simulink model "testmodel2017b"  (R2017b)
settings: Solver=FixedStepDiscrete  StartTime=0.0  StopTime=10000  FixedStep=srate  RelTol=1e-3
PreLoadFcn:
  | model_startup;
model workspace (MAT data in the model file):
  CD_IFBK_GAIN = Simulink.Parameter
  CD_IFBK_GAIN.Value = 0.00279947916667
  CD_IFBK_GAIN.DataType = 'single'
  CD_IFBK_GAIN.Dimensions = [1 1]
  CD_INTEGRATOR_RESET_I = Simulink.Parameter
  CD_INTEGRATOR_RESET_I.Value = 0.01
  CD_INTEGRATOR_RESET_I.DataType = 'single'
  CD_INTEGRATOR_RESET_I.Dimensions = [1 1]
  CD_PRECISION_REF_NOM = Simulink.Parameter
  CD_PRECISION_REF_NOM.Value = 511
  CD_PRECISION_REF_NOM.DataType = 'single'
  CD_PRECISION_REF_NOM.Dimensions = [1 1]
  CD_SOLENOID_RES = Simulink.Parameter
  CD_SOLENOID_RES.Value = 6.1803
  CD_SOLENOID_RES.DataType = 'single'
  CD_SOLENOID_RES.Dimensions = [1 1]
  CD_VBATTERY_GAIN = Simulink.Parameter
  CD_VBATTERY_GAIN.Value = 0.0293360157816
  CD_VBATTERY_GAIN.DataType = 'single'
  CD_VBATTERY_GAIN.Dimensions = [1 1]
  CD_VBATTERY_NOM = Simulink.Parameter
  CD_VBATTERY_NOM.Value = 13.5
  CD_VBATTERY_NOM.DataType = 'single'
  CD_VBATTERY_NOM.Dimensions = [1 1]
  OnPower = Simulink.Signal
  OnPower.DataType = 'boolean'
  OnPower.Dimensions = -1
  OnPower.DimensionsMode = 'auto'
  OnPower.Complexity = 'auto'
  OnPower.SampleTime = -1
  OnPower.SamplingMode = 'auto'
  numOutputs = 6
  srate = 0.01
undefined symbols (not defined in the file): CMD_INVERTER_GOTO_OPERATIONAL, CMD_INVERTER_GOTO_READY, CMD_INVERTER_GOTO_STOP, CMD_INVERTER_RUN_FWD, INVERTER_CONNECTED, INVERTER_OPERATIONAL, INVERTER_READY, INVERTER_RUN_FWD, INVERTER_STOP
libraries: simulink x8
CloseFcn:
  | model_end;
settings Model: Creator=cswenson  LastModifiedBy=mmaffeo
settings DataIOCC: SaveOutput=off  SaveTime=off
settings OptimizationCC: DefaultParameterBehavior=Inlined  InlineInvariantSignals=on  EnhancedBackFolding=on  PassReuseOutputArgsAs=Individual arguments  LifeSpan=inf  OptimizeBlockOrder=speed  DifferentSizesBufferReuse=on
settings DebuggingCC: SignalInfNanChecking=error  SignalRangeChecking=error  ReadBeforeWriteMsg=EnableAllAsError  WriteAfterWriteMsg=EnableAllAsError  WriteAfterReadMsg=EnableAllAsError  AlgebraicLoopMsg=error  ArtificialAlgebraicLoopMsg=error  SaveWithParameterizedLinksMsg=error  BlockPriorityViolationMsg=error  SolverPrmCheckMsg=error  InheritedTsInSrcMsg=error  SigSpecEnsureSampleTimeMsg=error  CheckMatrixSingularityMsg=error  IntegerOverflowMsg=error  ParameterUnderflowMsg=warning  ParameterTunabilityLossMsg=error  UnderSpecifiedDataTypeMsg=error  UnnecessaryDatatypeConvMsg=warning  VectorMatrixConversionMsg=error  FcnCallInpInsideContextMsg=warning  UnconnectedInputMsg=error  UnconnectedOutputMsg=error  UnconnectedLineMsg=error  SFcnCompatibilityMsg=error  UniqueDataStoreMsg=error  BusObjectLabelMismatch=error  RootOutportRequireBusObject=error  AssertControl=DisableAll  ModelReferenceIOMsg=error  ModelReferenceIOMismatchMessage=error  UnknownTsInhSupMsg=error  ModelReferenceDataLoggingMessage=error  StateNameClashWarn=warning  SFUnexpectedBacktrackingDiag=warning  SFNoUnconditionalDefaultTransitionDiag=warning  SFExecutionAtInitializationDiag=none
settings HardwareCC: ProdBitPerPointer=32  ProdBitPerSizeT=32  ProdBitPerPtrDiffT=32  ProdLargestAtomicInteger=Long  ProdLargestAtomicFloat=Double  ProdWordSize=32  ProdHWDeviceType=ARM Compatible->ARM Cortex  TargetBitPerPointer=64  TargetBitPerSizeT=64  TargetBitPerPtrDiffT=64  TargetLongLongMode=on  TargetIntDivRoundTo=Zero  TargetEndianess=LittleEndian  TargetWordSize=64  TargetHWDeviceType=MATLAB Host
settings ModelReferenceCC: PropagateSignalLabelsOutOfModel=off
settings SFSimCC: SimUserSources=SendMsgNow_Blank.cpp  SimUserIncludeDirs=functions  MATLABDynamicMemAlloc=off
settings SFSimCC: SimCustomHeaderCode=|
  | #include "SendMsgNow.h"
  | #define uint8_t unsigned char
settings RTWCC: SystemTargetFile=bobcat_ert.tlc  GenCodeOnly=on  GenerateMakefile=off  TemplateMakefile=ert_default_tmf  Description=Bobcat Embedded Target derived from RTW-EC  GenerateReport=on  RTWVerbose=off  IncludeHyperlinkInReport=on  LaunchReport=on  PortableWordSizes=on  TargetLang=C++  GenerateTraceInfo=on  GenerateTraceReport=on  GenerateTraceReportSl=on  GenerateTraceReportSf=on  GenerateTraceReportEml=on  GenerateCodeMetricsReport=on  GenerateCodeReplacementReport=on
settings RTWCC: CustomHeaderCode=|
  | #include "cdata.h"
  | #include "ap_can.h"
  | #include "SendMsgNow.h"
  | #include "ap_eeprom.h"
  | #include "ap_bservice_CAN04.h"
settings CodeAppCC: ForceParamTrailComments=on  IgnoreCustomStorageClasses=off  IgnoreTestpoints=on  MangleLength=4  StateflowObjectComments=on  InternalIdentifier=Classic  ReqsInCode=on
settings STFCustomTargetCC: MultiwordLength=256  IncludeMdlTerminateFcn=off  CombineOutputUpdateFcns=on  ERTCustomFileBanners=on  SupportNonFinite=off  SupportComplex=off  SupportNonInlinedSFcns=off  MATLABClassNameForMDSCustomization=Simulink.SoftwareTarget.ERTCustomization  GRTInterface=off  SystemTargetFile=bobcat_ert.tlc
settings ERTTargetCC: ParMdlRefBuildCompliant=off  CompOptLevelCompliant=off  ConcurrentExecutionCompliant=off  IncludeMdlTerminateFcn=off  SupportNonFinite=off  SupportComplex=off  SupportContinuousTime=on  RemoveResetFunc=off  ModelStepFunctionPrototypeControlCompliant=off  CPPClassGenCompliant=off  UseToolchainInfoCompliant=off  InlinedParameterPlacement=NonHierarchical  ERTSrcFileBannerTemplate=bobcat_ert_template.cgt  ERTHdrFileBannerTemplate=bobcat_ert_template.cgt  ERTDataSrcFileTemplate=bobcat_ert_template.cgt  ERTDataHdrFileTemplate=bobcat_ert_template.cgt  ERTCustomFileTemplate=bobcat_file_process.tlc  PreserveExpressionOrder=on  PreserveIfCondition=on  ConvertIfToSwitch=off  SuppressUnreachableDefaultCases=off
settings ConfigComp: CovScope=ReferencedModels  CovIncludeTopModel=off  CovMetricSettings=dw  CovHtmlReporting=on  CovSaveCumulativeToWorkspaceVar=on  CovSaveSingleToWorkspaceVar=on  CovExternalEMLEnable=off  CovSFcnEnable=off

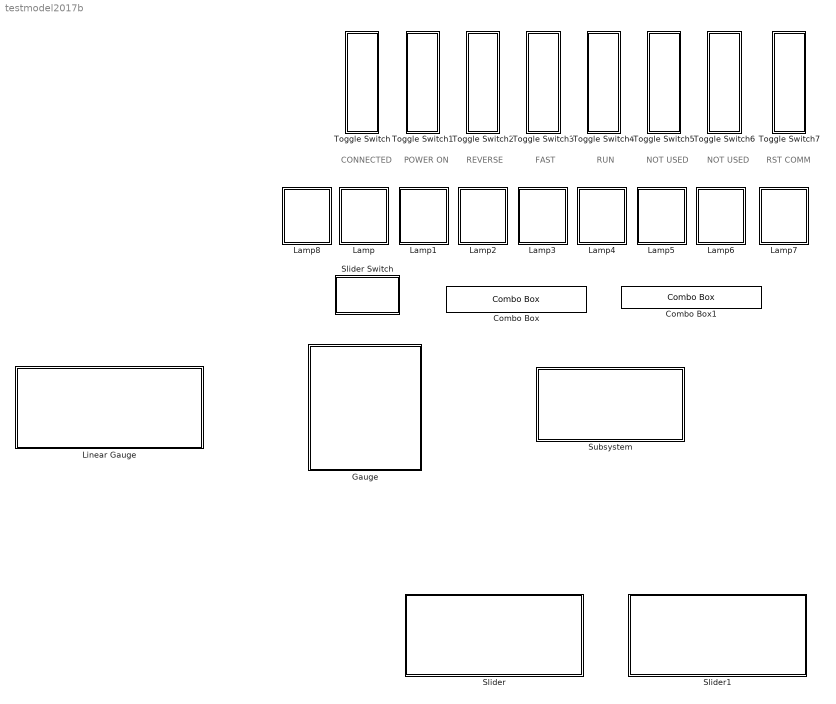
== system testmodel2017b ==
  note: CONNECTED
  note: POWER ON
  note: REVERSE
  note: FAST
  note: RST COMM
  note: RUN
  note: NOT USED
  note: NOT USED
  Combo Box : ComboBox  WebBlockId=8705  ModelName=testmodel2017b  LabelPosition=Top  ShowInitialText=on  SelectedLabel=connected
      settings: Values={{'stop', 'connected', 'operational', 'ready', 'run fwd', 'run rev'}, [0 1 2 3 4 5]}
  Combo Box1 : ComboBox  WebBlockId=8718  ModelName=testmodel2017b  LabelPosition=Hide  ShowInitialText=on  SelectedLabel=Go connected
      settings: Values={{'Go stop', 'Go connected', 'Go operational', 'Go ready', 'Run fwd', 'Run rev'}, [0 1 2 3 4 5]}
  Gauge : Subsystem  DialogController=hmiCreateDDGDialog  IsWebBlock=on  mask(MWDashboardBlock){webBlockId=ca701e44-4673-470a-9dd6-e67335b96dcc, webBlockType=circulargauge, ShowInLibBrowser=on, ShowInitialText=on, HMISrcModelName=testmodel2017b}
      mask prompts: webBlockId "WebBlock Id"; webBlockType "WebBlock Type"; HMISrcModelName "Source Model"
      mask help: SimulinkHMI:dialogs:CircularGaugeDialogDesc
      mask Help: helpview([docroot '/mapfiles/simulink.map'], 'hmi_gauge')
      mask Display:
      | if strcmp(get_param(bdroot(gcb),'BlockDiagramType'), 'library')
      |     image([(matlabroot) '/toolbox/simulink/hmi/icons/CircularGauge.png']);
      | end
  Lamp : Subsystem  DialogController=hmiCreateDDGDialog  IsWebBlock=on  mask(MWDashboardBlock){webBlockId=e5efdb02-b152-4998-b93d-c5098a951710, webBlockType=lamp, ShowInLibBrowser=on, ShowInitialText=on, HMISrcModelName=testmodel2017b}
      mask prompts: webBlockType "WebBlock Type"; HMISrcModelName "Source Model"
      mask help: SimulinkHMI:dialogs:LampDialogDesc
      mask Help: helpview([docroot '/mapfiles/simulink.map'], 'hmi_lamp')
      mask Display:
      | if strcmp(get_param(bdroot(gcb),'BlockDiagramType'), 'library')
      |     image([(matlabroot) '/toolbox/simulink/hmi/icons/Lamp.png']);
      | end
  Lamp1 : Subsystem  DialogController=hmiCreateDDGDialog  IsWebBlock=on  mask(MWDashboardBlock){webBlockId=63b4d971-4d5b-4e04-8404-41c9367548c4, webBlockType=lamp, ShowInLibBrowser=on, ShowInitialText=on, HMISrcModelName=testmodel2017b}
      mask prompts: webBlockType "WebBlock Type"; HMISrcModelName "Source Model"
      mask help: SimulinkHMI:dialogs:LampDialogDesc
      mask Help: helpview([docroot '/mapfiles/simulink.map'], 'hmi_lamp')
      mask Display:
      | if strcmp(get_param(bdroot(gcb),'BlockDiagramType'), 'library')
      |     image([(matlabroot) '/toolbox/simulink/hmi/icons/Lamp.png']);
      | end
  Lamp2 : Subsystem  DialogController=hmiCreateDDGDialog  IsWebBlock=on  mask(MWDashboardBlock){webBlockId=1f375b12-7dfa-43d5-91d3-510d879144cd, webBlockType=lamp, ShowInLibBrowser=on, ShowInitialText=on, HMISrcModelName=testmodel2017b}
      mask prompts: webBlockType "WebBlock Type"; HMISrcModelName "Source Model"
      mask help: SimulinkHMI:dialogs:LampDialogDesc
      mask Help: helpview([docroot '/mapfiles/simulink.map'], 'hmi_lamp')
      mask Display:
      | if strcmp(get_param(bdroot(gcb),'BlockDiagramType'), 'library')
      |     image([(matlabroot) '/toolbox/simulink/hmi/icons/Lamp.png']);
      | end
  Lamp3 : Subsystem  DialogController=hmiCreateDDGDialog  IsWebBlock=on  mask(MWDashboardBlock){webBlockId=32eb3db2-569b-4998-b9f3-c8386aa7fdc4, webBlockType=lamp, ShowInLibBrowser=on, ShowInitialText=on, HMISrcModelName=testmodel2017b}
      mask prompts: webBlockType "WebBlock Type"; HMISrcModelName "Source Model"
      mask help: SimulinkHMI:dialogs:LampDialogDesc
      mask Help: helpview([docroot '/mapfiles/simulink.map'], 'hmi_lamp')
      mask Display:
      | if strcmp(get_param(bdroot(gcb),'BlockDiagramType'), 'library')
      |     image([(matlabroot) '/toolbox/simulink/hmi/icons/Lamp.png']);
      | end
  Lamp4 : Subsystem  DialogController=hmiCreateDDGDialog  IsWebBlock=on  mask(MWDashboardBlock){webBlockId=7549cc86-a63f-4448-9fa5-76606dadb3b5, webBlockType=lamp, ShowInLibBrowser=on, ShowInitialText=on, HMISrcModelName=testmodel2017b}
      mask prompts: webBlockType "WebBlock Type"; HMISrcModelName "Source Model"
      mask help: SimulinkHMI:dialogs:LampDialogDesc
      mask Help: helpview([docroot '/mapfiles/simulink.map'], 'hmi_lamp')
      mask Display:
      | if strcmp(get_param(bdroot(gcb),'BlockDiagramType'), 'library')
      |     image([(matlabroot) '/toolbox/simulink/hmi/icons/Lamp.png']);
      | end
  Lamp5 : Subsystem  DialogController=hmiCreateDDGDialog  IsWebBlock=on  mask(MWDashboardBlock){webBlockId=152205e6-5cfd-45b8-b9ce-7b993e20bd51, webBlockType=lamp, ShowInLibBrowser=on, ShowInitialText=on, HMISrcModelName=testmodel2017b}
      mask prompts: webBlockType "WebBlock Type"; HMISrcModelName "Source Model"
      mask help: SimulinkHMI:dialogs:LampDialogDesc
      mask Help: helpview([docroot '/mapfiles/simulink.map'], 'hmi_lamp')
      mask Display:
      | if strcmp(get_param(bdroot(gcb),'BlockDiagramType'), 'library')
      |     image([(matlabroot) '/toolbox/simulink/hmi/icons/Lamp.png']);
      | end
  Lamp6 : Subsystem  DialogController=hmiCreateDDGDialog  IsWebBlock=on  mask(MWDashboardBlock){webBlockId=018165aa-a7d5-4652-b695-d8def093f8d2, webBlockType=lamp, ShowInLibBrowser=on, ShowInitialText=on, HMISrcModelName=testmodel2017b}
      mask prompts: webBlockType "WebBlock Type"; HMISrcModelName "Source Model"
      mask help: SimulinkHMI:dialogs:LampDialogDesc
      mask Help: helpview([docroot '/mapfiles/simulink.map'], 'hmi_lamp')
      mask Display:
      | if strcmp(get_param(bdroot(gcb),'BlockDiagramType'), 'library')
      |     image([(matlabroot) '/toolbox/simulink/hmi/icons/Lamp.png']);
      | end
  Lamp7 : Subsystem  DialogController=hmiCreateDDGDialog  IsWebBlock=on  mask(MWDashboardBlock){webBlockId=cac63575-c101-4763-9fa7-36335908d754, webBlockType=lamp, ShowInLibBrowser=on, ShowInitialText=on, HMISrcModelName=testmodel2017b}
      mask prompts: webBlockType "WebBlock Type"; HMISrcModelName "Source Model"
      mask help: SimulinkHMI:dialogs:LampDialogDesc
      mask Help: helpview([docroot '/mapfiles/simulink.map'], 'hmi_lamp')
      mask Display:
      | if strcmp(get_param(bdroot(gcb),'BlockDiagramType'), 'library')
      |     image([(matlabroot) '/toolbox/simulink/hmi/icons/Lamp.png']);
      | end
  Lamp8 : Subsystem  DialogController=hmiCreateDDGDialog  IsWebBlock=on  mask(MWDashboardBlock){webBlockId=dd506db5-93af-464d-82af-439ee47e3a28, webBlockType=lamp, ShowInLibBrowser=on, ShowInitialText=on, HMISrcModelName=testmodel2017b}
      mask prompts: webBlockType "WebBlock Type"; HMISrcModelName "Source Model"
      mask help: SimulinkHMI:dialogs:LampDialogDesc
      mask Help: helpview([docroot '/mapfiles/simulink.map'], 'hmi_lamp')
      mask Display:
      | if strcmp(get_param(bdroot(gcb),'BlockDiagramType'), 'library')
      |     image([(matlabroot) '/toolbox/simulink/hmi/icons/Lamp.png']);
      | end
  Linear Gauge : Subsystem  DialogController=hmiCreateDDGDialog  IsWebBlock=on  mask(MWDashboardBlock){webBlockId=7f63c228-2e19-4776-af30-abd338e55317, webBlockType=lineargauge, ShowInLibBrowser=on, ShowInitialText=on, HMISrcModelName=testmodel2017b}
      mask prompts: webBlockId "WebBlock Id"; webBlockType "WebBlock Type"; HMISrcModelName "Source Model"
      mask help: SimulinkHMI:dialogs:LinearGaugeDialogDesc
      mask Help: helpview([docroot '/mapfiles/simulink.map'], 'hmi_linear_gauge')
      mask Display:
      | if strcmp(get_param(bdroot(gcb),'BlockDiagramType'), 'library')
      |     image([(matlabroot) '/toolbox/simulink/hmi/icons/LinearGauge.png']);
      | end
  Slider : Subsystem  DialogController=hmiCreateDDGDialog  IsWebBlock=on  mask(MWDashboardBlock){webBlockId=fa958995-471b-4ba4-bec5-340cf4a0c4a4, webBlockType=slider, ShowInLibBrowser=on, ShowInitialText=on, HMISrcModelName=testmodel2017b}
      mask prompts: webBlockId "WebBlock Id"; webBlockType "WebBlock Type"; HMISrcModelName "Source Model"
      mask help: SimulinkHMI:dialogs:SliderDialogDesc
      mask Help: helpview([docroot '/mapfiles/simulink.map'], 'hmi_slider')
      mask Display:
      | if strcmp(get_param(bdroot(gcb),'BlockDiagramType'), 'library')
      |     image([(matlabroot) '/toolbox/simulink/hmi/icons/Slider.png']);
      | end
  Slider Switch : Subsystem  DialogController=hmiCreateDDGDialog  IsWebBlock=on  mask(MWDashboardBlock){webBlockId=162e49f7-e18d-4260-a1e1-ddee9463ac9c, webBlockType=sliderswitch, ShowInLibBrowser=on, ShowInitialText=on, HMISrcModelName=testmodel2017b}
      mask prompts: webBlockId "WebBlock Id"; webBlockType "WebBlock Type"; HMISrcModelName "Source Model"
      mask help: SimulinkHMI:dialogs:SwitchDialogDesc
      mask Help: helpview([docroot '/mapfiles/simulink.map'], 'hmi_slider_switch')
      mask Display:
      | if strcmp(get_param(bdroot(gcb),'BlockDiagramType'), 'library')
      |     image([(matlabroot) '/toolbox/simulink/hmi/icons/SliderSwitch.png']);
      | end
  Slider1 : Subsystem  DialogController=hmiCreateDDGDialog  IsWebBlock=on  mask(MWDashboardBlock){webBlockId=517096a1-4060-40ba-819b-9a3d476b2f75, webBlockType=slider, ShowInLibBrowser=on, ShowInitialText=on, HMISrcModelName=testmodel2017b}
      mask prompts: webBlockId "WebBlock Id"; webBlockType "WebBlock Type"; HMISrcModelName "Source Model"
      mask help: SimulinkHMI:dialogs:SliderDialogDesc
      mask Help: helpview([docroot '/mapfiles/simulink.map'], 'hmi_slider')
      mask Display:
      | if strcmp(get_param(bdroot(gcb),'BlockDiagramType'), 'library')
      |     image([(matlabroot) '/toolbox/simulink/hmi/icons/Slider.png']);
      | end
  Subsystem : Subsystem
  Toggle Switch : Subsystem  DialogController=hmiCreateDDGDialog  IsWebBlock=on  mask(MWDashboardBlock){webBlockId=8c672047-e032-446a-86cd-f25ef30b8805, webBlockType=toggleswitch, ShowInLibBrowser=on, ShowInitialText=on, HMISrcModelName=testmodel2017b}
      mask prompts: webBlockId "WebBlock Id"; webBlockType "WebBlock Type"; HMISrcModelName "Source Model"
      mask help: SimulinkHMI:dialogs:SwitchDialogDesc
      mask Help: helpview([docroot '/mapfiles/simulink.map'], 'hmi_toggle_switch')
      mask Display:
      | if strcmp(get_param(bdroot(gcb),'BlockDiagramType'), 'library')
      |     image([(matlabroot) '/toolbox/simulink/hmi/icons/ToggleSwitch.png']);
      | end
  Toggle Switch1 : Subsystem  DialogController=hmiCreateDDGDialog  IsWebBlock=on  mask(MWDashboardBlock){webBlockId=0751683d-a109-4dd3-9882-3b03258bbb54, webBlockType=toggleswitch, ShowInLibBrowser=on, ShowInitialText=on, HMISrcModelName=testmodel2017b}
      mask prompts: webBlockId "WebBlock Id"; webBlockType "WebBlock Type"; HMISrcModelName "Source Model"
      mask help: SimulinkHMI:dialogs:SwitchDialogDesc
      mask Help: helpview([docroot '/mapfiles/simulink.map'], 'hmi_toggle_switch')
      mask Display:
      | if strcmp(get_param(bdroot(gcb),'BlockDiagramType'), 'library')
      |     image([(matlabroot) '/toolbox/simulink/hmi/icons/ToggleSwitch.png']);
      | end
  Toggle Switch2 : Subsystem  DialogController=hmiCreateDDGDialog  IsWebBlock=on  mask(MWDashboardBlock){webBlockId=8ca877d7-0c1a-426d-a4f9-a2827789716f, webBlockType=toggleswitch, ShowInLibBrowser=on, ShowInitialText=on, HMISrcModelName=testmodel2017b}
      mask prompts: webBlockId "WebBlock Id"; webBlockType "WebBlock Type"; HMISrcModelName "Source Model"
      mask help: SimulinkHMI:dialogs:SwitchDialogDesc
      mask Help: helpview([docroot '/mapfiles/simulink.map'], 'hmi_toggle_switch')
      mask Display:
      | if strcmp(get_param(bdroot(gcb),'BlockDiagramType'), 'library')
      |     image([(matlabroot) '/toolbox/simulink/hmi/icons/ToggleSwitch.png']);
      | end
  Toggle Switch3 : Subsystem  DialogController=hmiCreateDDGDialog  IsWebBlock=on  mask(MWDashboardBlock){webBlockId=da84f3e4-9ca8-45fc-be02-ca49a032c9c0, webBlockType=toggleswitch, ShowInLibBrowser=on, ShowInitialText=on, HMISrcModelName=testmodel2017b}
      mask prompts: webBlockId "WebBlock Id"; webBlockType "WebBlock Type"; HMISrcModelName "Source Model"
      mask help: SimulinkHMI:dialogs:SwitchDialogDesc
      mask Help: helpview([docroot '/mapfiles/simulink.map'], 'hmi_toggle_switch')
      mask Display:
      | if strcmp(get_param(bdroot(gcb),'BlockDiagramType'), 'library')
      |     image([(matlabroot) '/toolbox/simulink/hmi/icons/ToggleSwitch.png']);
      | end
  Toggle Switch4 : Subsystem  DialogController=hmiCreateDDGDialog  IsWebBlock=on  mask(MWDashboardBlock){webBlockId=9eeb4cfb-cb7f-4c09-9385-0d917563cd64, webBlockType=toggleswitch, ShowInLibBrowser=on, ShowInitialText=on, HMISrcModelName=testmodel2017b}
      mask prompts: webBlockId "WebBlock Id"; webBlockType "WebBlock Type"; HMISrcModelName "Source Model"
      mask help: SimulinkHMI:dialogs:SwitchDialogDesc
      mask Help: helpview([docroot '/mapfiles/simulink.map'], 'hmi_toggle_switch')
      mask Display:
      | if strcmp(get_param(bdroot(gcb),'BlockDiagramType'), 'library')
      |     image([(matlabroot) '/toolbox/simulink/hmi/icons/ToggleSwitch.png']);
      | end
  Toggle Switch5 : Subsystem  DialogController=hmiCreateDDGDialog  IsWebBlock=on  mask(MWDashboardBlock){webBlockId=0c1a0a0b-1c4b-493f-aa89-501afe314834, webBlockType=toggleswitch, ShowInLibBrowser=on, ShowInitialText=on, HMISrcModelName=testmodel2017b}
      mask prompts: webBlockId "WebBlock Id"; webBlockType "WebBlock Type"; HMISrcModelName "Source Model"
      mask help: SimulinkHMI:dialogs:SwitchDialogDesc
      mask Help: helpview([docroot '/mapfiles/simulink.map'], 'hmi_toggle_switch')
      mask Display:
      | if strcmp(get_param(bdroot(gcb),'BlockDiagramType'), 'library')
      |     image([(matlabroot) '/toolbox/simulink/hmi/icons/ToggleSwitch.png']);
      | end
  Toggle Switch6 : Subsystem  DialogController=hmiCreateDDGDialog  IsWebBlock=on  mask(MWDashboardBlock){webBlockId=cf9357e9-b879-40ce-aca0-e0c1ce0f2806, webBlockType=toggleswitch, ShowInLibBrowser=on, ShowInitialText=on, HMISrcModelName=testmodel2017b}
      mask prompts: webBlockId "WebBlock Id"; webBlockType "WebBlock Type"; HMISrcModelName "Source Model"
      mask help: SimulinkHMI:dialogs:SwitchDialogDesc
      mask Help: helpview([docroot '/mapfiles/simulink.map'], 'hmi_toggle_switch')
      mask Display:
      | if strcmp(get_param(bdroot(gcb),'BlockDiagramType'), 'library')
      |     image([(matlabroot) '/toolbox/simulink/hmi/icons/ToggleSwitch.png']);
      | end
  Toggle Switch7 : Subsystem  DialogController=hmiCreateDDGDialog  IsWebBlock=on  mask(MWDashboardBlock){webBlockId=bd6f0e80-1dc1-4bd1-a44d-bbc0d96f943f, webBlockType=toggleswitch, ShowInLibBrowser=on, ShowInitialText=on, HMISrcModelName=testmodel2017b}
      mask prompts: webBlockId "WebBlock Id"; webBlockType "WebBlock Type"; HMISrcModelName "Source Model"
      mask help: SimulinkHMI:dialogs:SwitchDialogDesc
      mask Help: helpview([docroot '/mapfiles/simulink.map'], 'hmi_toggle_switch')
      mask Display:
      | if strcmp(get_param(bdroot(gcb),'BlockDiagramType'), 'library')
      |     image([(matlabroot) '/toolbox/simulink/hmi/icons/ToggleSwitch.png']);
      | end

== system testmodel2017b/Gauge ==

== system testmodel2017b/Lamp ==

== system testmodel2017b/Lamp1 ==

== system testmodel2017b/Lamp2 ==

== system testmodel2017b/Lamp3 ==

== system testmodel2017b/Lamp4 ==

== system testmodel2017b/Lamp5 ==

== system testmodel2017b/Lamp6 ==

== system testmodel2017b/Lamp7 ==

== system testmodel2017b/Lamp8 ==

== system testmodel2017b/Linear Gauge ==

== system testmodel2017b/Slider ==

== system testmodel2017b/Slider Switch ==

== system testmodel2017b/Slider1 ==

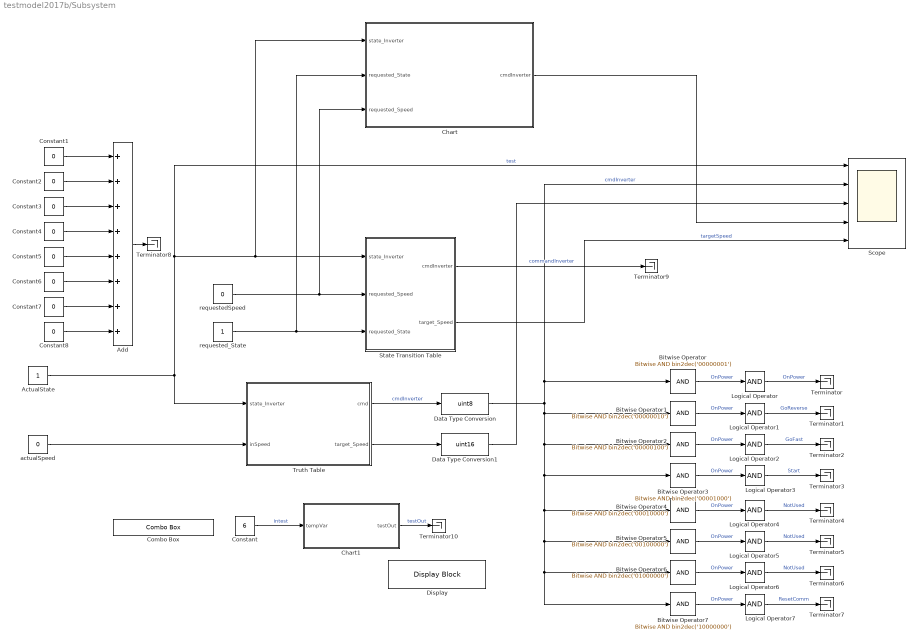
== system testmodel2017b/Subsystem ==
  ActualState : Constant  OutDataTypeStr=uint8
  Add : Sum  Inputs=++++++++  OutDataTypeStr=uint8
  Bitwise Operator : simulink/Logic and Bit Operations/Bitwise Operator  logicop=AND  UseBitMask=on  BitMask=bin2dec('00000001')  BitMaskRealWorld=Stored Integer
  Bitwise Operator1 : simulink/Logic and Bit Operations/Bitwise Operator  logicop=AND  UseBitMask=on  BitMask=bin2dec('00000010')  BitMaskRealWorld=Stored Integer
  Bitwise Operator2 : simulink/Logic and Bit Operations/Bitwise Operator  logicop=AND  UseBitMask=on  BitMask=bin2dec('00000100')  BitMaskRealWorld=Stored Integer
  Bitwise Operator3 : simulink/Logic and Bit Operations/Bitwise Operator  logicop=AND  UseBitMask=on  BitMask=bin2dec('00001000')  BitMaskRealWorld=Stored Integer
  Bitwise Operator4 : simulink/Logic and Bit Operations/Bitwise Operator  logicop=AND  UseBitMask=on  BitMask=bin2dec('00010000')  BitMaskRealWorld=Stored Integer
  Bitwise Operator5 : simulink/Logic and Bit Operations/Bitwise Operator  logicop=AND  UseBitMask=on  BitMask=bin2dec('00100000')  BitMaskRealWorld=Stored Integer
  Bitwise Operator6 : simulink/Logic and Bit Operations/Bitwise Operator  logicop=AND  UseBitMask=on  BitMask=bin2dec('01000000')  BitMaskRealWorld=Stored Integer
  Bitwise Operator7 : simulink/Logic and Bit Operations/Bitwise Operator  logicop=AND  UseBitMask=on  BitMask=bin2dec('10000000')  BitMaskRealWorld=Stored Integer
  Chart : Stateflow chart  TreatAsAtomicUnit=on
  Chart1 : Stateflow chart  TreatAsAtomicUnit=on
  Combo Box : ComboBox  WebBlockId=8732  ModelName=testmodel2017b  LabelPosition=Hide  ShowInitialText=on  SelectedLabel=6
      settings: Values={{'0', '1', '2', '3', '4', '5', '6'}, [0 1 2 3 4 5 6]}
  Constant : Constant  Value=6
  Constant{1..8} (8 alike) : Constant  Value=0
  Data Type Conversion : DataTypeConversion  OutDataTypeStr=uint8
  Data Type Conversion1 : DataTypeConversion  OutDataTypeStr=uint16
  Display : DisplayBlock  WebBlockId=8735  ModelName=testmodel2017b  LabelPosition=Hide  ShowInitialText=on  ShowFormattedStrings=off  Format=long  Alignment=Center
  Logical Operator{,1..7} (8 alike) : Logic  Inputs=1  AllPortsSameDT=off  OutDataTypeStr=boolean
  Scope : Scope  NumInputPorts=5
  State Transition Table : State Transition Table  TreatAsAtomicUnit=on
  Terminator{,1..10} (11 alike) : Terminator
  Truth Table : Truth Table  TreatAsAtomicUnit=on
  actualSpeed : Constant  Value=0  OutDataTypeStr=uint16
  requestedSpeed : Constant  Value=0  OutDataTypeStr=uint16
  requested_State : Constant  OutDataTypeStr=uint8
  wires:
  ActualState/1 -> Chart/1(state_Inverter), State Transition Table/1(state_Inverter), Scope/1, Truth Table/1(state_Inverter)  "test"
  Constant1/1 -> Add/1
  Constant7/1 -> Add/7
  Constant5/1 -> Add/5
  Constant6/1 -> Add/6
  Constant8/1 -> Add/8
  Constant4/1 -> Add/4
  Constant2/1 -> Add/2
  Constant3/1 -> Add/3
  Logical Operator/1 -> Terminator/1  "OnPower"
  Logical Operator1/1 -> Terminator1/1  "GoReverse"
  Logical Operator4/1 -> Terminator4/1  "NotUsed"
  Logical Operator5/1 -> Terminator5/1  "NotUsed"
  Logical Operator6/1 -> Terminator6/1  "NotUsed"
  Logical Operator7/1 -> Terminator7/1  "ResetComm"
  Data Type Conversion/1 -> Bitwise Operator7/1, Bitwise Operator6/1, Bitwise Operator5/1, Bitwise Operator4/1, Bitwise Operator3/1, Bitwise Operator2/1, Bitwise Operator1/1, Bitwise Operator/1, Scope/2  "cmdInverter"
  Bitwise Operator/1 -> Logical Operator/1  "OnPower"
  Bitwise Operator1/1 -> Logical Operator1/1  "OnPower"
  Bitwise Operator2/1 -> Logical Operator2/1  "OnPower"
  Bitwise Operator3/1 -> Logical Operator3/1  "OnPower"
  Logical Operator2/1 -> Terminator2/1  "GoFast"
  Logical Operator3/1 -> Terminator3/1  "Start"
  Bitwise Operator7/1 -> Logical Operator7/1  "OnPower"
  Bitwise Operator4/1 -> Logical Operator4/1  "OnPower"
  Bitwise Operator6/1 -> Logical Operator6/1  "OnPower"
  Bitwise Operator5/1 -> Logical Operator5/1  "OnPower"
  Data Type Conversion1/1 -> Scope/3
  Add/1 -> Terminator8/1
  actualSpeed/1 -> Truth Table/2(inSpeed)
  Truth Table/1(cmd) -> Data Type Conversion/1  "cmdInverter"
  Truth Table/2(target_Speed) -> Data Type Conversion1/1
  requested_State/1 -> Chart/2(requested_State), State Transition Table/3(requested_State)
  State Transition Table/1(cmdInverter) -> Terminator9/1  "commandInverter"
  State Transition Table/2(target_Speed) -> Scope/5  "targetSpeed"
  requestedSpeed/1 -> Chart/3(requested_Speed), State Transition Table/2(requested_Speed)
  Chart/1(cmdInverter) -> Scope/4
  Constant/1 -> Chart1/1(tempVar)  "intest"
  Chart1/1(testOut) -> Terminator10/1  "testOut"

== system testmodel2017b/Toggle Switch ==

== system testmodel2017b/Toggle Switch1 ==

== system testmodel2017b/Toggle Switch2 ==

== system testmodel2017b/Toggle Switch3 ==

== system testmodel2017b/Toggle Switch4 ==

== system testmodel2017b/Toggle Switch5 ==

== system testmodel2017b/Toggle Switch6 ==

== system testmodel2017b/Toggle Switch7 ==

== stateflow chart testmodel2017b/Subsystem/Chart1 ==
  state prova
    du:testOut = 0;
  state prova2
    du:testOut = 6;
  state prova1
    du:testOut = 2;
  (default) -> prova
  prova2 -> prova [order 2] : [tempVar == 6]{testOut = 7}
  prova -> prova2 [order 1] : [tempVar == 2]{testOut = 8}
  prova -> prova1 [order 2] : [tempVar == 1]{testOut = 1}
  prova1 -> prova [order 2] : [tempVar == 5]{testOut = 3}
  prova2 -> prova1 [order 1] : [tempVar == 3]{testOut = 5}
  prova1 -> prova2 [order 1] : [tempVar == 4]{testOut = 4}
  data: testOut output double; tempVar input double

== matlab function testmodel2017b/Subsystem/Truth Table ==
  data: state_Inverter input uint8; cmd output double; target_Speed output double; inSpeed input uint16
function [cmd, target_Speed] = fcn(state_Inverter, inSpeed)

aVarTruthTableCondition_1 = false;
aVarTruthTableCondition_2 = false;
aVarTruthTableCondition_3 = false;
aVarTruthTableCondition_4 = false;
aVarTruthTableCondition_5 = false;


% Example condition 1

aVarTruthTableCondition_1 = logical(state_Inverter == 0);

% Example condition 2

aVarTruthTableCondition_2 = logical(state_Inverter == 1);


aVarTruthTableCondition_3 = logical(state_Inverter == 2);


aVarTruthTableCondition_4 = logical(state_Inverter == 3);


aVarTruthTableCondition_5 = logical(state_Inverter == 4);

if (aVarTruthTableCondition_1 && ~aVarTruthTableCondition_2 && ~aVarTruthTableCondition_3 && ~aVarTruthTableCondition_4 && ~aVarTruthTableCondition_5)
    aFcnTruthTableAction_1();
elseif (aVarTruthTableCondition_1 && aVarTruthTableCondition_2 && ~aVarTruthTableCondition_3 && ~aVarTruthTableCondition_4 && ~aVarTruthTableCondition_5)
    aFcnTruthTableAction_2();
elseif (aVarTruthTableCondition_1 && aVarTruthTableCondition_2 && aVarTruthTableCondition_3 && aVarTruthTableCondition_4 && ~aVarTruthTableCondition_5)
    aFcnTruthTableAction_3();
elseif (aVarTruthTableCondition_1 && aVarTruthTableCondition_2 && aVarTruthTableCondition_3 && aVarTruthTableCondition_4 && aVarTruthTableCondition_5)
    aFcnTruthTableAction_3();
else % Default
    aFcnTruthTableAction_3();
end

function aFcnTruthTableAction_1()

% Example action 1 called from D1 & D2 column in condition table

cmd = 0
target_Speed = 0

function aFcnTruthTableAction_2()

% Example action 2 called from D3 column in condition table

cmd = 0
target_Speed = 0

function aFcnTruthTableAction_3()


cmd = 0
target_Speed = 0

== stateflow chart testmodel2017b/Subsystem/Chart ==
  state STOP
  state GOTO_OPERATIONAL
    en:cmdInverter = 0;
  state OPERATIONAL
  (default) -> STOP
  STOP -> GOTO_OPERATIONAL [order 2] : [state_Inverter == INVERTER_STOP]{cmdInverter = 3}
  STOP -> OPERATIONAL [order 1] : [state_Inverter  >= INVERTER_OPERATIONAL]
  OPERATIONAL -> STOP : [state_Inverter  < INVERTER_CONNECTED]
  GOTO_OPERATIONAL -> OPERATIONAL
  data: state_Inverter input; requested_State input; requested_Speed input; INVERTER_STOP parameter; INVERTER_CONNECTED parameter; INVERTER_RUN_FWD parameter; INVERTER_READY parameter; CMD_INVERTER_GOTO_OPERATIONAL parameter; INVERTER_OPERATIONAL parameter; cmdInverter output double

== stateflow chart testmodel2017b/Subsystem/State Transition Table ==
  state STOP
    state GOTO_OPERATIONAL
    (default) -> GOTO_OPERATIONAL
    GOTO_OPERATIONAL -> (junction 130) : [requested_State  >=INVERTER_CONNECTED]
        | {cmdInverter = CMD_INVERTER_GOTO_OPERATIONAL}
    (junction 130) -> GOTO_OPERATIONAL
  state OPERATIONAL
    state GOTO_READY
    (default) -> GOTO_READY
    GOTO_READY -> (junction 153) : [requested_State  >=INVERTER_READY]
        | {cmdInverter = CMD_INVERTER_GOTO_READY}
    (junction 153) -> GOTO_READY
  state READY
  state RUN
  (default) -> STOP
  STOP -> (junction 123) [order 2] : [requested_State  < INVERTER_CONNECTED ]
      | {cmdInverter = CMD_INVERTER_GOTO_STOP}
  (junction 123) -> STOP
  STOP -> OPERATIONAL [order 1] : [state_Inverter  >= INVERTER_CONNECTED]
  OPERATIONAL -> STOP [order 3] : [requested_State  < INVERTER_READY ]
      | {cmdInverter = CMD_INVERTER_GOTO_OPERATIONAL}
  OPERATIONAL -> (junction 105) [order 2] : [requested_State  >= INVERTER_CONNECTED]
      | {cmdInverter = CMD_INVERTER_GOTO_READY}
  (junction 105) -> OPERATIONAL
  OPERATIONAL -> READY [order 1] : [state_Inverter  >= INVERTER_READY ]
  READY -> OPERATIONAL [order 3] : [requested_State  < INVERTER_RUN_FWD ]
      | {cmdInverter = CMD_INVERTER_GOTO_OPERATIONAL}
  READY -> (junction 108) [order 2] : [requested_State  == INVERTER_RUN_FWD ]
      | {cmdInverter = CMD_INVERTER_RUN_FWD}
  (junction 108) -> READY
  READY -> RUN [order 1] : [state_Inverter  >= INVERTER_RUN_FWD & requested_Speed >= 0]
  RUN -> READY [order 2] : [requested_Speed == 0]
      | {cmdInverter = CMD_INVERTER_GOTO_READY}
  RUN -> (junction 49) [order 1] : [requested_Speed > 0]
      | {target_Speed = requested_Speed}
  (junction 49) -> RUN
  data: state_Inverter input uint8; INVERTER_CONNECTED parameter; INVERTER_READY parameter; INVERTER_RUN_FWD parameter; requested_Speed input uint16; requested_State input uint8; cmdInverter output uint8; target_Speed output uint16; CMD_INVERTER_RUN_FWD parameter; INVERTER_STOP parameter; CMD_INVERTER_GOTO_READY parameter; CMD_INVERTER_GOTO_OPERATIONAL parameter; CMD_INVERTER_GOTO_STOP parameter
